simulink model "TST_AdvancedStateflowLoops3"  (Simulink 7.4)
settings: Solver=FixedStepDiscrete  StartTime=0.0  StopTime=10.0  FixedStep=0.02  RelTol=1e-3
settings Model: Creator=kharthforeign  LastModifiedBy=kharthforeign  BufferReuse=off
settings DataIOCC: SaveOutput=off  SignalLogging=off  SaveTime=off
settings OptimizationCC: BlockReduction=off  ConditionallyExecuteInputs=off  OptimizeBlockIOStorage=off  BufferReuse=off  ExpressionFolding=off  LocalBlockOutputs=off  InitFltsAndDblsToZero=on

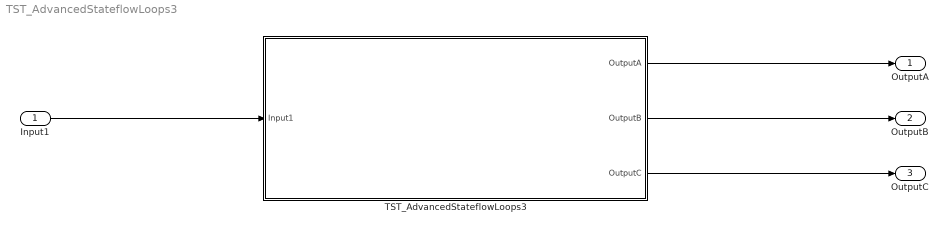
== system TST_AdvancedStateflowLoops3 ==
  Input1 : Inport  DataType=uint32  OutDataType=fixdt(1, 16)  OutScaling=2^0  OutDataTypeStr=uint32  BusOutputAsStruct=on
  TST_AdvancedStateflowLoops3 : Subsystem  TreatAsAtomicUnit=on
  OutputA : Outport  PortDimensions=1  DataType=double  OutDataType=fixdt(1, 16)  OutScaling=2^0  OutDataTypeStr=double
  OutputB : Outport  Port=2  PortDimensions=1  DataType=double  OutDataType=Enum: DIL_VmmGsFcsCommandsMessage_LatApModeCmd  OutDataTypeStr=double
  OutputC : Outport  Port=3  PortDimensions=1  DataType=double  OutDataType=fixdt(1, 16)  OutScaling=2^0  OutDataTypeStr=double
  wires:
  Input1/1 -> TST_AdvancedStateflowLoops3/1(Input1)
  TST_AdvancedStateflowLoops3/1(OutputA) -> OutputA/1
  TST_AdvancedStateflowLoops3/2(OutputB) -> OutputB/1
  TST_AdvancedStateflowLoops3/3(OutputC) -> OutputC/1

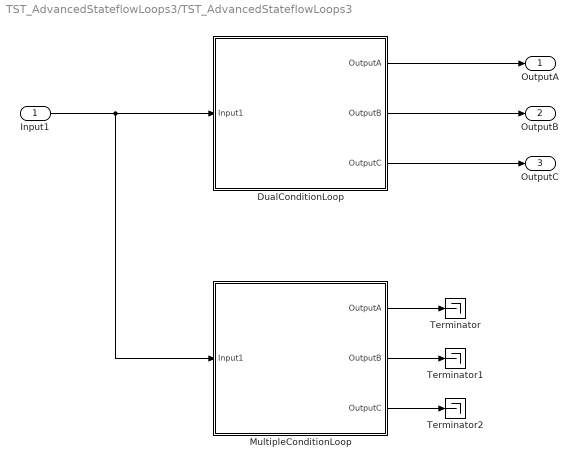
== system TST_AdvancedStateflowLoops3/TST_AdvancedStateflowLoops3 ==
  Input1 : Inport  DataType=uint32  OutDataType=fixdt(1, 16)  OutScaling=2^0  OutDataTypeStr=uint32  BusOutputAsStruct=on
  DualConditionLoop : Stateflow chart
  MultipleConditionLoop : Stateflow chart
  Terminator : Terminator
  Terminator1 : Terminator
  Terminator2 : Terminator
  OutputA : Outport  PortDimensions=1  DataType=double  OutDataType=fixdt(1, 16)  OutScaling=2^0  OutDataTypeStr=double
  OutputB : Outport  Port=2  PortDimensions=1  DataType=double  OutDataType=Enum: DIL_VmmGsFcsCommandsMessage_LatApModeCmd  OutDataTypeStr=double
  OutputC : Outport  Port=3  PortDimensions=1  DataType=double  OutDataType=fixdt(1, 16)  OutScaling=2^0  OutDataTypeStr=double
  wires:
  DualConditionLoop/1(OutputA) -> OutputA/1
  DualConditionLoop/2(OutputB) -> OutputB/1
  DualConditionLoop/3(OutputC) -> OutputC/1
  Input1/1 -> DualConditionLoop/1(Input1), MultipleConditionLoop/1(Input1)
  MultipleConditionLoop/1(OutputA) -> Terminator/1
  MultipleConditionLoop/2(OutputB) -> Terminator1/1
  MultipleConditionLoop/3(OutputC) -> Terminator2/1

== stateflow chart TST_AdvancedStateflowLoops3/MultipleConditionLoop ==
  note: This flowgraph demonstrates three single-transition loops.
      | Semantically they all are part of the same repeat statement.
  (junction 5) -> (junction 4) [order 4] : {OutputC = 99.0}
  (junction 5) -> (junction 5) [order 2] : [B]{OutputB += 2.0}
  (default) -> (junction 5)
  (junction 5) -> (junction 5) [order 1] : [A]{OutputA += 1.0}
  (junction 5) -> (junction 5) [order 3] : [C]{OutputC += 3.0}
  data: Input1 input uint32; OutputA output double =1; OutputB output double =2; OutputC output double =3; Local local uint32 =0; A local boolean; B local boolean; C local boolean; D local boolean

== stateflow chart TST_AdvancedStateflowLoops3/DualConditionLoop ==
  state StateX
  note: This flowgraph demonstrates two indiviual loops that are semantically joined.
      | Because they have the same loop source/destination junction, they are
      | part of the same repeat statement.
  (junction 25) -> StateX [order 3] : {OutputC = 7.0}
  (junction 25) -> (junction 24) [order 2] : [B]
  (default) -> (junction 25)
  (junction 24) -> (junction 25) : {OutputB += 2.0}
  (junction 25) -> (junction 26) [order 1] : [A]
  (junction 26) -> (junction 25) : {OutputA += 2.0}
  data: Input1 input uint32; OutputA output double =1; OutputB output double =2; OutputC output double =3; Local local uint32 =0; A local boolean; B local boolean; C local boolean; D local boolean
